simulink model "controle_proporcional_onoff_pid"  (R2013a)
settings: Solver=ode3  StartTime=0.0  StopTime=inf  FixedStep=0.01  RelTol=1e-3
undefined symbols (not defined in the file or in its folder): analoginput, analogoutput
libraries: daqlib x2, simulink x2, simulink_extras x1
settings Model: Creator=paulo.costa  LastModifiedBy=paulo.costa

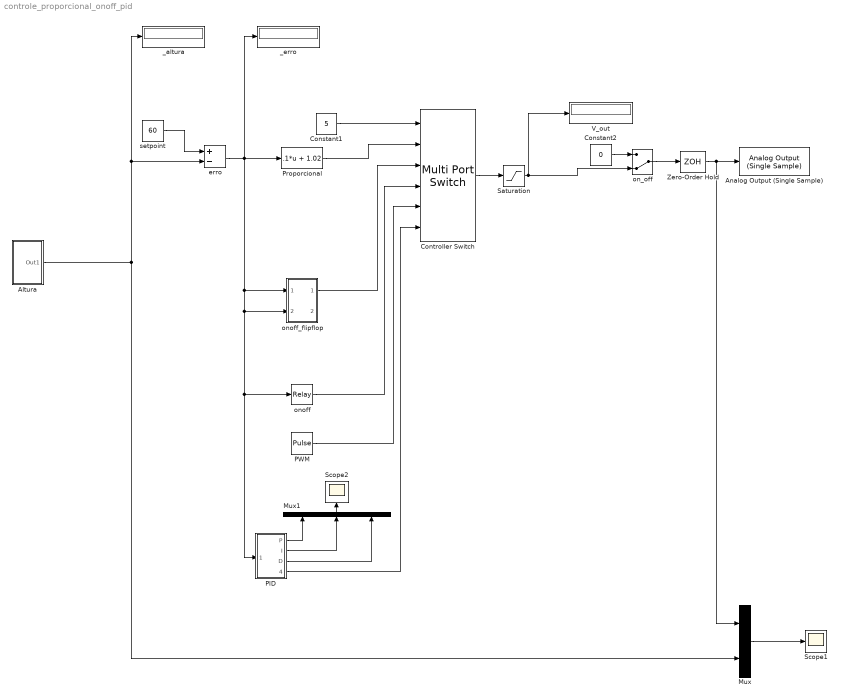
== system controle_proporcional_onoff_pid ==
  Altura : Subsystem
  Analog Output (Single Sample) : daqlib/Analog Output (Single Sample)  DeviceMenu=nidaq Dev1 (USB-6009)  Device=nidaq Dev1 (USB-6009)  ObjConstructor=analogoutput('nidaq','Dev1')  NChannelsSelected=1  Channels=1$0$$1$0$#0$1$$1$0$#  NPorts=1 for all hardware channels
  Constant1 : Constant  Value=5
  Constant2 : Constant  Value=0
  Controller Switch : MultiPortSwitch  Inputs=5
  Mux : Mux  Inputs=2
  Mux1 : Mux  Inputs=3
  PID : Subsystem
  PWM : DiscretePulseGenerator  PulseType=Time based  Amplitude=5  Period=1  PulseWidth=10
  "Proporcional " : Fcn  Expr=.1*u + 1.02
  Saturation : Saturate  UpperLimit=5  LowerLimit=0
  Scope1 : Scope
      settings: TimeRange=10  YMin=0  YMax=65
  Scope2 : Scope
      settings: YMin=-1.25  YMax=2.25  SaveName=ScopeData2
  V_out : Display
      settings: Decimation=5
  Zero-Order Hold : ZeroOrderHold  SampleTime=.01
  _altura : Display
  _erro : Display
  erro : Sum  Inputs=+-
  on_off : ManualSwitch  CurrentSetting=0
  onoff : Relay  OnSwitchValue=10  OffSwitchValue=-10  OnOutputValue=5  OffOutputValue=1
  onoff_flipflop : Subsystem
  setpoint : Constant  Value=60
  wires:
  erro/1 -> "Proporcional "/1, _erro/1, onoff_flipflop/1(In1), onoff/1, PID/1(In1), onoff_flipflop/2(In2)
  Zero-Order Hold/1 -> Mux/1, Analog Output (Single Sample)/1
  setpoint/1 -> erro/1
  Mux/1 -> Scope1/1
  PWM/1 -> Controller Switch/5
  onoff/1 -> Controller Switch/4
  Constant1/1 -> Controller Switch/1
  Constant2/1 -> on_off/1
  on_off/1 -> Zero-Order Hold/1
  Controller Switch/1 -> Saturation/1
  "Proporcional "/1 -> Controller Switch/2
  PID/1(P) -> Mux1/1
  PID/2(I) -> Mux1/2
  PID/3(D) -> Mux1/3
  Mux1/1 -> Scope2/1
  PID/4(PID) -> Controller Switch/6
  onoff_flipflop/1(Out1) -> Controller Switch/3
  Altura/1(Out1) -> erro/2, _altura/1, Mux/2
  Saturation/1 -> on_off/2, V_out/1

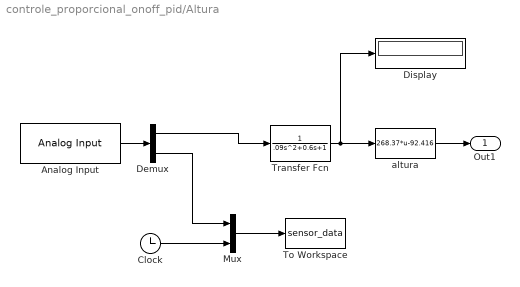
== system controle_proporcional_onoff_pid/Altura ==
  Analog Input : daqlib/Analog Input  AcqMode=0  DeviceMenu=nidaq Dev1 (USB-6009)  Device=nidaq Dev1 (USB-6009)  ObjConstructor=analoginput('nidaq','Dev1')  SampleRate=200  ActualRate=200  SamplesPerFrame=2  InputType=SingleEnded  NChannelsSelected=1  Channels=1$0$$2$#0$1$$2$#0$2$$2$#0$3$$2$#0$4$$2$#0$5$$2$#0$6$$2$#0$7$$2$#  NPorts=1 for all hardware channels  DataType=double
      settings: SignalType=Sample-based
  Clock : Clock
  Demux : Demux  Outputs=2
  Display : Display
  Mux : Mux  Inputs=2
  To Workspace : ToWorkspace  VariableName=sensor_data  SampleTime=-1
  Transfer Fcn : TransferFcn  Denominator=[.09 0.6 1]
  altura : Fcn  Expr=268.37*u-92.416
  Out1 : Outport
  wires:
  altura/1 -> Out1/1
  Analog Input/1 -> Demux/1
  Demux/2 -> Mux/1
  Transfer Fcn/1 -> Display/1, altura/1
  Demux/1 -> Transfer Fcn/1
  Mux/1 -> To Workspace/1
  Clock/1 -> Mux/2

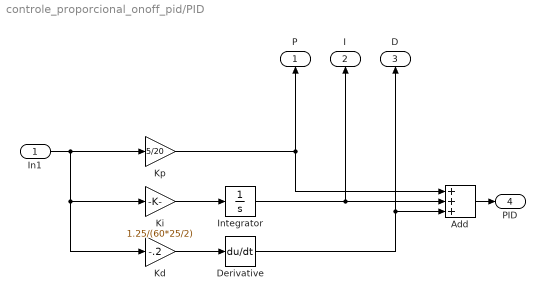
== system controle_proporcional_onoff_pid/PID ==
  In1 : Inport
  Add : Sum  Inputs=+++
  Derivative : Derivative
  Integrator : Integrator
  Kd : Gain  Gain=-.2
  Ki : Gain  Gain=1.25/(60*25/2)
  Kp : Gain  Gain=5/20
  P : Outport
  I : Outport  Port=2
  D : Outport  Port=3
  PID : Outport  Port=4
  wires:
  Ki/1 -> Integrator/1
  In1/1 -> Kd/1, Ki/1, Kp/1
  Derivative/1 -> D/1, Add/3
  Add/1 -> PID/1
  Integrator/1 -> I/1, Add/2
  Kp/1 -> P/1, Add/1
  Kd/1 -> Derivative/1

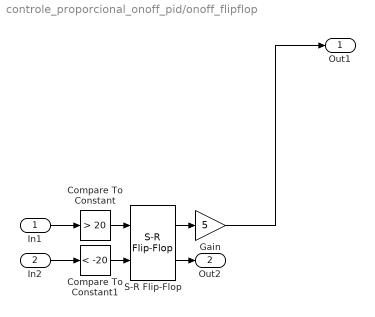
== system controle_proporcional_onoff_pid/onoff_flipflop ==
  In1 : Inport
  In2 : Inport  Port=2
  Compare To Constant : simulink/Logic and Bit Operations/Compare To Constant  relop=>  const=20  OutDataTypeStr=boolean
  Compare To Constant1 : simulink/Logic and Bit Operations/Compare To Constant  relop=<  const=-20  OutDataTypeStr=boolean
  Gain : Gain  Gain=5
  S-R Flip-Flop : simulink_extras/Flip Flops/S-R Flip-Flop  initial_condition=0
  Out1 : Outport
  Out2 : Outport  Port=2
  wires:
  Compare To Constant/1 -> S-R Flip-Flop/1
  S-R Flip-Flop/1 -> Gain/1
  Compare To Constant1/1 -> S-R Flip-Flop/2
  Gain/1 -> Out1/1
  In2/1 -> Compare To Constant1/1
  In1/1 -> Compare To Constant/1
  S-R Flip-Flop/2 -> Out2/1
